simulink model "Logging"  (Simulink 9.1)
settings: Solver=VariableStepAuto  StartTime=0.0  StopTime=10.0  RelTol=1e-3
libraries: F_Line_block x59
settings Model: LogicAnalyzerSignalOrdering=8bf68fb7-e9c2-472a-a2d5-0b6182d7556c  Creator=dongw  LastModifiedBy=dongw
settings DataIOCC: SaveFormat=Dataset
settings OptimizationCC: LifeSpan=auto
settings DebuggingCC: UnderspecifiedInitializationDetection=Simplified  MergeDetectMultiDrivingBlocksExec=error  SFUnexpectedBacktrackingDiag=error  SFNoUnconditionalDefaultTransitionDiag=error  SFExecutionAtInitializationDiag=warning
settings HardwareCC: ProdBitPerPointer=64  ProdBitPerSizeT=64  ProdBitPerPtrDiffT=64  ProdLargestAtomicFloat=Float  ProdIntDivRoundTo=Zero  ProdEndianess=LittleEndian  ProdWordSize=64  ProdHWDeviceType=Intel->x86-64 (Windows64)
settings ModelReferenceCC: PropagateSignalLabelsOutOfModel=on
settings CodeAppCC: StateflowObjectComments=off
settings GRTTargetCC: TargetLangStandard=C99 (ISO)  CombineOutputUpdateFcns=on  GRTInterface=off
settings ConfigComp: CovMetricSettings=dwe  CovHtmlReporting=off  CovSaveCumulativeToWorkspaceVar=off  CovSaveSingleToWorkspaceVar=off  CovExternalEMLEnable=on

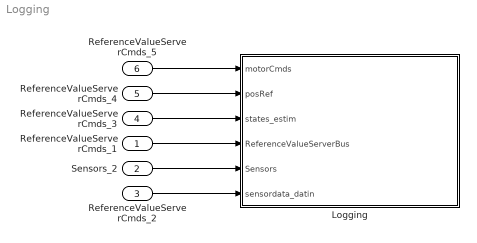
== system Logging ==
  ReferenceValueServerCmds_1 : Inport  OutDataTypeStr=Bus: CommandBus
  Sensors_2 : Inport  Port=2  OutDataTypeStr=Bus: SensorsBus  BusOutputAsStruct=on
  ReferenceValueServerCmds_2 : Inport  Port=3  OutDataTypeStr=Bus: CommandBus
  ReferenceValueServerCmds_3 : Inport  Port=4  OutDataTypeStr=Bus: CommandBus
  ReferenceValueServerCmds_4 : Inport  Port=5  OutDataTypeStr=Bus: CommandBus
  ReferenceValueServerCmds_5 : Inport  Port=6  OutDataTypeStr=Bus: CommandBus
  Logging : Subsystem  TreatAsAtomicUnit=on
      settings: RTWFcnNameOpts=Use subsystem name
  wires:
  ReferenceValueServerCmds_4/1 -> Logging/2(posRef)
  ReferenceValueServerCmds_3/1 -> Logging/3(states_estim)
  Sensors_2/1 -> Logging/5(Sensors)
  ReferenceValueServerCmds_1/1 -> Logging/4(ReferenceValueServerBus)
  ReferenceValueServerCmds_2/1 -> Logging/6(sensordata_datin)
  ReferenceValueServerCmds_5/1 -> Logging/1(motorCmds)

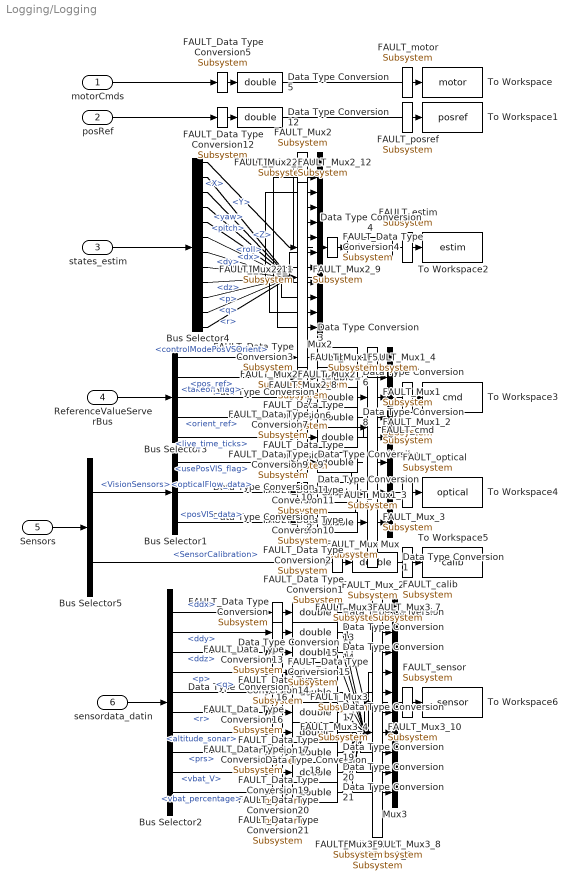
== system Logging/Logging ==
  motorCmds : Inport
  posRef : Inport  Port=2
  states_estim : Inport  Port=3  OutDataTypeStr=Bus: statesEstim_t  BusOutputAsStruct=on
  ReferenceValueServerBus : Inport  Port=4  OutDataTypeStr=Bus: CommandBus  BusOutputAsStruct=on
  Sensors : Inport  Port=5  OutDataTypeStr=Bus: SensorsBus
  sensordata_datin : Inport  Port=6  OutDataTypeStr=Bus: sensordata_t
  Bus Selector1 : BusSelector  OutputSignals=usePosVIS_flag,opticalFlow_data,posVIS_data
  Bus Selector2 : BusSelector  OutputSignals=ddx,ddy,ddz,p,q,r,altitude_sonar,prs,vbat_V,vbat_percentage
  Bus Selector3 : BusSelector  OutputSignals=controlModePosVSOrient,pos_ref,takeoff_flag,orient_ref,live_time_ticks
  Bus Selector4 : BusSelector  OutputSignals=X,Y,Z,yaw,pitch,roll,dx,dy,dz,p,q,r
  Bus Selector5 : BusSelector  OutputSignals=VisionSensors,SensorCalibration
  Data Type Conversion{,1..21} (22 alike) : DataTypeConversion  OutDataTypeStr=double
  FAULT_Data Type Conversion{,1..21} (22 alike) : F_Line_block/Subsystem
  Mux : Mux  Inputs=3
  FAULT_Mux{,1..3} (4 alike) : F_Line_block/Subsystem
  FAULT_Mux_2 : F_Line_block/Subsystem
  FAULT_Mux_3 : F_Line_block/Subsystem
  Mux1 : Mux  Inputs=5
  FAULT_Mux1_{2..5} (4 alike) : F_Line_block/Subsystem
  Mux2 : Mux  Inputs=12
  FAULT_Mux2_{2..12} (11 alike) : F_Line_block/Subsystem
  Mux3 : Mux  Inputs=10
  FAULT_Mux3_{2..10} (9 alike) : F_Line_block/Subsystem
  To Workspace : ToWorkspace  VariableName=motor  SaveFormat=Structure With Time  SampleTime=-1
  FAULT_motor : F_Line_block/Subsystem
  To Workspace1 : ToWorkspace  VariableName=posref  SaveFormat=Structure With Time  SampleTime=-1
  FAULT_posref : F_Line_block/Subsystem
  To Workspace2 : ToWorkspace  VariableName=estim  SaveFormat=Structure With Time  SampleTime=-1
  FAULT_estim : F_Line_block/Subsystem
  To Workspace3 : ToWorkspace  VariableName=cmd  SaveFormat=Structure With Time  SampleTime=-1
  FAULT_cmd : F_Line_block/Subsystem
  To Workspace4 : ToWorkspace  VariableName=optical  SaveFormat=Structure With Time  SampleTime=-1
  FAULT_optical : F_Line_block/Subsystem
  To Workspace5 : ToWorkspace  VariableName=calib  SaveFormat=Structure With Time  SampleTime=-1
  FAULT_calib : F_Line_block/Subsystem
  To Workspace6 : ToWorkspace  VariableName=sensor  SaveFormat=Structure With Time  SampleTime=-1
  FAULT_sensor : F_Line_block/Subsystem
  wires:
  Bus Selector3/1 -> FAULT_Data Type Conversion3/1  "<controlModePosVSOrient>"
  FAULT_Data Type Conversion3/1 -> Data Type Conversion3/1
  Bus Selector3/3 -> FAULT_Data Type Conversion7/1  "<takeoff_flag>"
  FAULT_Data Type Conversion7/1 -> Data Type Conversion7/1
  Bus Selector3/4 -> FAULT_Data Type Conversion8/1  "<orient_ref>"
  FAULT_Data Type Conversion8/1 -> Data Type Conversion8/1
  Bus Selector3/5 -> FAULT_Data Type Conversion9/1  "<live_time_ticks>"
  FAULT_Data Type Conversion9/1 -> Data Type Conversion9/1
  ReferenceValueServerBus/1 -> Bus Selector3/1
  Bus Selector3/2 -> FAULT_Data Type Conversion6/1  "<pos_ref>"
  FAULT_Data Type Conversion6/1 -> Data Type Conversion6/1
  sensordata_datin/1 -> Bus Selector2/1
  Bus Selector2/1 -> FAULT_Data Type Conversion/1  "<ddx>"
  FAULT_Data Type Conversion/1 -> Data Type Conversion/1
  Sensors/1 -> Bus Selector5/1
  Bus Selector1/1 -> FAULT_Data Type Conversion11/1  "<usePosVIS_flag>"
  FAULT_Data Type Conversion11/1 -> Data Type Conversion11/1
  Bus Selector1/2 -> FAULT_Data Type Conversion10/1  "<opticalFlow_data>"
  FAULT_Data Type Conversion10/1 -> Data Type Conversion10/1
  Bus Selector1/3 -> FAULT_Data Type Conversion2/1  "<posVIS_data>"
  FAULT_Data Type Conversion2/1 -> Data Type Conversion2/1
  Data Type Conversion1/1 -> To Workspace5/1
  Bus Selector5/2 -> FAULT_Data Type Conversion1/1  "<SensorCalibration>"
  FAULT_Data Type Conversion1/1 -> Data Type Conversion1/1
  Mux/1 -> To Workspace4/1
  Data Type Conversion4/1 -> To Workspace2/1
  motorCmds/1 -> FAULT_Data Type Conversion5/1
  FAULT_Data Type Conversion5/1 -> Data Type Conversion5/1
  Data Type Conversion5/1 -> To Workspace/1
  Mux1/1 -> To Workspace3/1
  states_estim/1 -> Bus Selector4/1
  Mux2/1 -> FAULT_Data Type Conversion4/1
  FAULT_Data Type Conversion4/1 -> Data Type Conversion4/1
  Bus Selector4/4 -> FAULT_Mux2_4/1  "<yaw>"
  FAULT_Mux2_4/1 -> Mux2/4
  Bus Selector4/6 -> FAULT_Mux2_6/1  "<roll>"
  FAULT_Mux2_6/1 -> Mux2/6
  Bus Selector4/5 -> FAULT_Mux2_5/1  "<pitch>"
  FAULT_Mux2_5/1 -> Mux2/5
  Bus Selector4/9 -> FAULT_Mux2_9/1  "<dz>"
  FAULT_Mux2_9/1 -> Mux2/9
  Bus Selector4/7 -> FAULT_Mux2_7/1  "<dx>"
  FAULT_Mux2_7/1 -> Mux2/7
  Bus Selector4/8 -> FAULT_Mux2_8/1  "<dy>"
  FAULT_Mux2_8/1 -> Mux2/8
  Bus Selector4/10 -> FAULT_Mux2_10/1  "<p>"
  FAULT_Mux2_10/1 -> Mux2/10
  Bus Selector4/12 -> FAULT_Mux2_12/1  "<r>"
  FAULT_Mux2_12/1 -> Mux2/12
  Bus Selector4/2 -> FAULT_Mux2_2/1  "<Y>"
  FAULT_Mux2_2/1 -> Mux2/2
  Bus Selector4/11 -> FAULT_Mux2_11/1  "<q>"
  FAULT_Mux2_11/1 -> Mux2/11
  Bus Selector4/3 -> FAULT_Mux2_3/1  "<Z>"
  FAULT_Mux2_3/1 -> Mux2/3
  Bus Selector4/1 -> FAULT_Mux2/1  "<X>"
  FAULT_Mux2/1 -> Mux2/1
  Data Type Conversion3/1 -> FAULT_Mux1/1
  FAULT_Mux1/1 -> Mux1/1
  Data Type Conversion6/1 -> FAULT_Mux1_2/1
  FAULT_Mux1_2/1 -> Mux1/2
  Data Type Conversion7/1 -> FAULT_Mux1_3/1
  FAULT_Mux1_3/1 -> Mux1/3
  Data Type Conversion8/1 -> FAULT_Mux1_4/1
  FAULT_Mux1_4/1 -> Mux1/4
  Data Type Conversion9/1 -> FAULT_Mux1_5/1
  FAULT_Mux1_5/1 -> Mux1/5
  Data Type Conversion2/1 -> FAULT_Mux_3/1
  FAULT_Mux_3/1 -> Mux/3
  Data Type Conversion10/1 -> FAULT_Mux_2/1
  FAULT_Mux_2/1 -> Mux/2
  Data Type Conversion11/1 -> FAULT_Mux/1
  FAULT_Mux/1 -> Mux/1
  posRef/1 -> FAULT_Data Type Conversion12/1
  FAULT_Data Type Conversion12/1 -> Data Type Conversion12/1
  Data Type Conversion12/1 -> To Workspace1/1
  Bus Selector2/2 -> FAULT_Data Type Conversion13/1  "<ddy>"
  FAULT_Data Type Conversion13/1 -> Data Type Conversion13/1
  Bus Selector2/3 -> FAULT_Data Type Conversion14/1  "<ddz>"
  FAULT_Data Type Conversion14/1 -> Data Type Conversion14/1
  Bus Selector2/4 -> FAULT_Data Type Conversion15/1  "<p>"
  FAULT_Data Type Conversion15/1 -> Data Type Conversion15/1
  Bus Selector2/5 -> FAULT_Data Type Conversion16/1  "<q>"
  FAULT_Data Type Conversion16/1 -> Data Type Conversion16/1
  Bus Selector2/6 -> FAULT_Data Type Conversion17/1  "<r>"
  FAULT_Data Type Conversion17/1 -> Data Type Conversion17/1
  Bus Selector2/7 -> FAULT_Data Type Conversion18/1  "<altitude_sonar>"
  FAULT_Data Type Conversion18/1 -> Data Type Conversion18/1
  Bus Selector2/8 -> FAULT_Data Type Conversion19/1  "<prs>"
  FAULT_Data Type Conversion19/1 -> Data Type Conversion19/1
  Bus Selector2/9 -> FAULT_Data Type Conversion20/1  "<vbat_V>"
  FAULT_Data Type Conversion20/1 -> Data Type Conversion20/1
  Bus Selector2/10 -> FAULT_Data Type Conversion21/1  "<vbat_percentage>"
  FAULT_Data Type Conversion21/1 -> Data Type Conversion21/1
  Data Type Conversion/1 -> FAULT_Mux3/1
  FAULT_Mux3/1 -> Mux3/1
  Data Type Conversion13/1 -> FAULT_Mux3_2/1
  FAULT_Mux3_2/1 -> Mux3/2
  Data Type Conversion14/1 -> FAULT_Mux3_3/1
  FAULT_Mux3_3/1 -> Mux3/3
  Data Type Conversion15/1 -> FAULT_Mux3_4/1
  FAULT_Mux3_4/1 -> Mux3/4
  Data Type Conversion16/1 -> FAULT_Mux3_5/1
  FAULT_Mux3_5/1 -> Mux3/5
  Data Type Conversion17/1 -> FAULT_Mux3_6/1
  FAULT_Mux3_6/1 -> Mux3/6
  Data Type Conversion18/1 -> FAULT_Mux3_7/1
  FAULT_Mux3_7/1 -> Mux3/7
  Data Type Conversion19/1 -> FAULT_Mux3_8/1
  FAULT_Mux3_8/1 -> Mux3/8
  Data Type Conversion20/1 -> FAULT_Mux3_9/1
  FAULT_Mux3_9/1 -> Mux3/9
  Data Type Conversion21/1 -> FAULT_Mux3_10/1
  FAULT_Mux3_10/1 -> Mux3/10
  Mux3/1 -> To Workspace6/1
  Bus Selector5/1 -> Bus Selector1/1  "<VisionSensors>"
